simulink model "sepic_2"  (Simulink 7.4)
settings: Solver=ode23tb  StartTime=0.0  StopTime=.01  MaxStep=.01/Fswitch  RelTol=1e-3
InitFcn:
  | clc
  | Fswitch=330e3;
  | Comp_Tau=1e-8;
  | Vset=3.3;
  | Iout=1;
  | Rload=Vset/Iout;
  | Imax=2.5;
  | Iload=Imax-Iout;
  | Tload =5e-3;
  | FET_Ron=8e-3;
  | FET_Snub=1e3;
  | L1=4.6e-6;
  | L1_R = .005;
  | L2=L1;
  | L2_R=L1_R;
  | Cs=10e-6;
  | ESR_cs=.01;
  | Cout=140e-6;
  | ESR_out=4.8e-3;
  | Vfwd_Diode=0.25;
  | R_Diode=0.1;
libraries: powerlib x14, simulink x2, simulink_extras x1
settings Model: Creator=Dick  LastModifiedBy=dbenson  SimulationMode=accelerator
settings SolverCC: SolverResetMethod=Robust

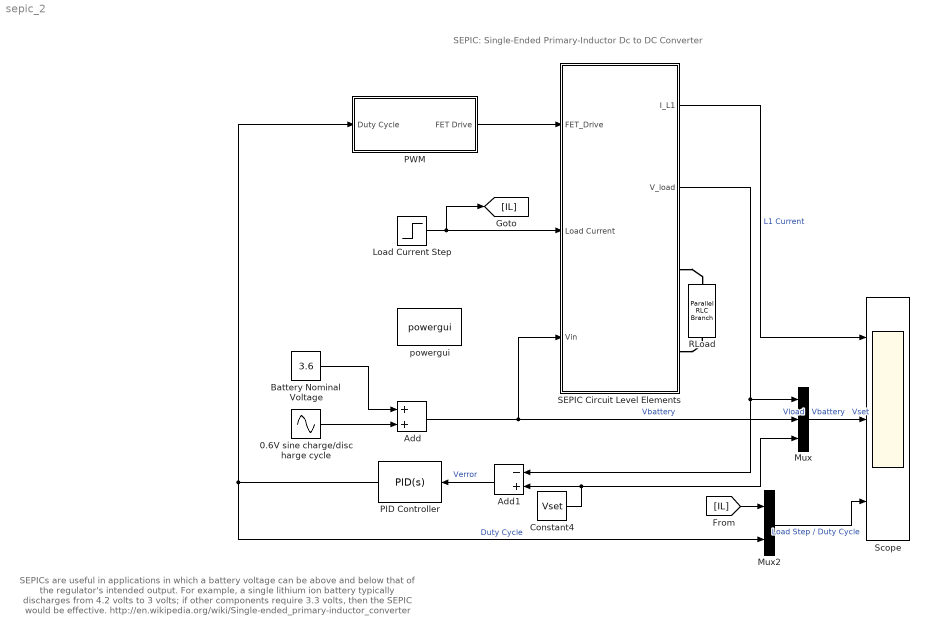
== system sepic_2 ==
  note: SEPICs are useful in applications in which a battery voltage  can be above and below that of the regulator's intended output.
      |  For example, a single lithium ion battery typically discharges from 4.2 volts to 3 volts; if other components require 3.3 volts,
      | then the SEPIC would be effective.
      |
      | http://en.wikipedia.org/wiki/Single-ended_primary-inductor_converter
  note: SEPIC: Single-Ended Primary-Inductor Dc to DC Converter
  0.6V sine charge/discharge cycle : Sin  Amplitude=.6  Bias=0  Frequency=2*pi*100  Phase=0  Samples=10  SampleTime=0  Offset=0
  Add : Sum  OutDataType=fixdt(1, 16)  OutScaling=2^-10
  Add1 : Sum  Inputs=-+  OutDataType=fixdt(1, 16)  OutScaling=2^-10
  Battery Nominal Voltage : Constant  Value=3.6  OutDataType=fixdt(1, 16)  OutScaling=2^0
  Constant4 : Constant  Value=Vset  OutDataType=fixdt(1, 16)  OutScaling=2^0
  Load Current Step : Step  Time=Tload  After=Iload  SampleTime=0
  Mux : Mux  Inputs=3
  Mux2 : Mux  Inputs=2
  PID Controller : simulink/Continuous/PID Controller  DialogController=pidpack.PIDConfig.pidDDGCreate  DialogControllerArgs=DataTag0  SystemSampleTime=-1  Controller=PID  TimeDomain=Continuous-time  SampleTime=1  IntegratorMethod=Forward Euler  FilterMethod=Forward Euler  Form=Parallel  P=.1  I=1000  D=0  N=100  InitialConditionSource=internal  InitialConditionForIntegrator=0  InitialConditionForFilter=0  ExternalReset=none  LimitOutput=off  UpperSaturationLimit=inf  LowerSaturationLimit=-inf  LinearizeAsGain=off  AntiWindupMode=none  Kb=1  TrackingMode=off  Kt=1  PParamMin=[]  PParamMax=[]  IParamMin=[]  IParamMax=[]  DParamMin=[]  DParamMax=[]  NParamMin=[]  NParamMax=[]  KbParamMin=[]  KbParamMax=[]  KtParamMin=[]  KtParamMax=[]  POutMin=[]  POutMax=[]  IOutMin=[]  IOutMax=[]  DOutMin=[]  DOutMax=[]  NOutMin=[]  NOutMax=[]  KbOutMin=[]  KbOutMax=[]  KtOutMin=[]  KtOutMax=[]  IntegratorOutMin=[]  IntegratorOutMax=[]  FilterOutMin=[]  FilterOutMax=[]  SumOutMin=[]  SumOutMax=[]  SumI1OutMin=[]  SumI1OutMax=[]  SumI2OutMin=[]  SumI2OutMax=[]  SumI3OutMin=[]  SumI3OutMax=[]  SumDOutMin=[]  SumDOutMax=[]  SaturationOutMin=[]  SaturationOutMax=[]  IntegratorContinuousStateAttributes=''  IntegratorStateMustResolveToSignalObject=off  IntegratorRTWStateStorageClass=Auto  FilterContinuousStateAttributes=''  FilterStateMustResolveToSignalObject=off  FilterRTWStateStorageClass=Auto
  PWM : Subsystem  mask{Fsw=Fswitch, Tau=Comp_Tau}
      mask prompts: Fsw "Switch Frequency"; Tau "Comparitor Time Constant"
  RLoad : powerlib/Elements/Parallel RLC Branch  DialogController=POWERSYS.PowerSysDialog  PhysicalDomain=powersysdomain  SubClassName=unknown  LeftPortType=p1  RightPortType=p1  LConnTagsString=a  RConnTagsString=__new0  BranchType=R  Resistance=Rload  Inductance=1e-3  SetiL0=off  InitialCurrent=0  Capacitance=1e-6  Setx0=off  InitialVoltage=0  Measurements=None
  SEPIC Circuit Level Elements : Subsystem
  Scope : Scope  NumInputPorts=3
      settings: TimeRange=0.01  YMin=-10~0~-0.3  YMax=10~5~1.7  MaxDataPoints=1e6
  powergui : powerlib/powergui  Priority=1  SystemSampleTime=-1  SimulationMode=Continuous  SampleTime=50e-6  frequency=60  SPID=off  DisableSnubberDevices=off  DisableRonSwitches=off  DisableVfSwitches=off  SwTol=0  Interpol=off  frequencyindice=0  echomessages=off  HookPort=off  DisplayEquations=off  FunctionMessages=off  EnableUseOfTLC=off  x0status=blocks  RestoreLinks=warning  Frange=[0:2:500]  Ylog=off  Xlog=on  ShowGrid=off  save=off  variable=ZData  ZoomFFT=on  StartTime=0.0  cycles=1  DisplayStyle=1  fundamental=60  FreqAxis=off  MaxFrequency=1000  frequencyindicesteady=1  RmsSteady=1  display=off  Ts=0  methode=off
  wires:
  PWM/1(FET Drive) -> SEPIC Circuit Level Elements/1(FET_Drive)
  0.6V sine charge/discharge cycle/1 -> Add/2
  Load Current Step/1 -> SEPIC Circuit Level Elements/2(Load Current), [IL]
  SEPIC Circuit Level Elements/2(V_load) -> Add1/1, Mux/1
  Add1/1 -> PID Controller/1  "Verror"
  Constant4/1 -> Add1/2, Mux/3
  PID Controller/1 -> PWM/1(Duty Cycle), Mux2/2  "Duty Cycle"
  Add/1 -> SEPIC Circuit Level Elements/3(Vin), Mux/2  "Vbattery"
  Battery Nominal Voltage/1 -> Add/1
  Mux/1 -> Scope/2  "Vload   Vbattery   Vset"
  SEPIC Circuit Level Elements/1(I_L1) -> Scope/1  "L1 Current"
  Mux2/1 -> Scope/3  "Load Step / Duty Cycle"
  [IL] -> Mux2/1
  connections:
  SEPIC Circuit Level Elements/RConn1 -- RLoad/LConn1
  SEPIC Circuit Level Elements/RConn2 -- RLoad/RConn1

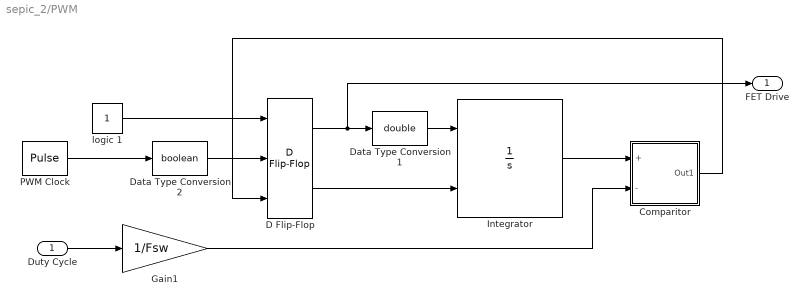
== system sepic_2/PWM ==
  Duty Cycle : Inport  OutDataType=sfix(16)  OutScaling=2^0
  Comparitor : Subsystem
  D Flip-Flop : simulink_extras/Flip Flops/D Flip-Flop  SystemSampleTime=-1
  Data Type Conversion1 : DataTypeConversion  OutDataTypeMode=double  OutDataType=fixdt(1,16,16)  OutDataTypeStr=double  SaturateOnIntegerOverflow=on
  Data Type Conversion2 : DataTypeConversion  OutDataTypeMode=boolean  OutDataType=fixdt(1,16,16)  OutDataTypeStr=boolean  SaturateOnIntegerOverflow=on
  Gain1 : Gain  Gain=1/Fsw  ParameterDataType=fixdt(1, 16)  ParameterScaling=2^0  OutDataType=fixdt(1, 16)  OutScaling=2^0
  Integrator : Integrator  ExternalReset=level
  PWM Clock : DiscretePulseGenerator  PulseType=Time based  Amplitude=1  Period=1/Fsw  PulseWidth=50  PhaseDelay=0  SampleTime=1
  logic 1 : Constant  OutDataTypeMode=boolean  OutDataType=sfix(16)  OutScaling=2^0  OutDataTypeStr=boolean
  FET Drive : Outport  OutDataType=sfix(16)  OutScaling=2^0
  wires:
  D Flip-Flop/2 -> Integrator/2
  logic 1/1 -> D Flip-Flop/1
  Integrator/1 -> Comparitor/1(+)
  D Flip-Flop/1 -> FET Drive/1, Data Type Conversion1/1
  Comparitor/1(Out1) -> D Flip-Flop/3
  Data Type Conversion2/1 -> D Flip-Flop/2
  Data Type Conversion1/1 -> Integrator/1
  Duty Cycle/1 -> Gain1/1
  Gain1/1 -> Comparitor/2(-)
  PWM Clock/1 -> Data Type Conversion2/1

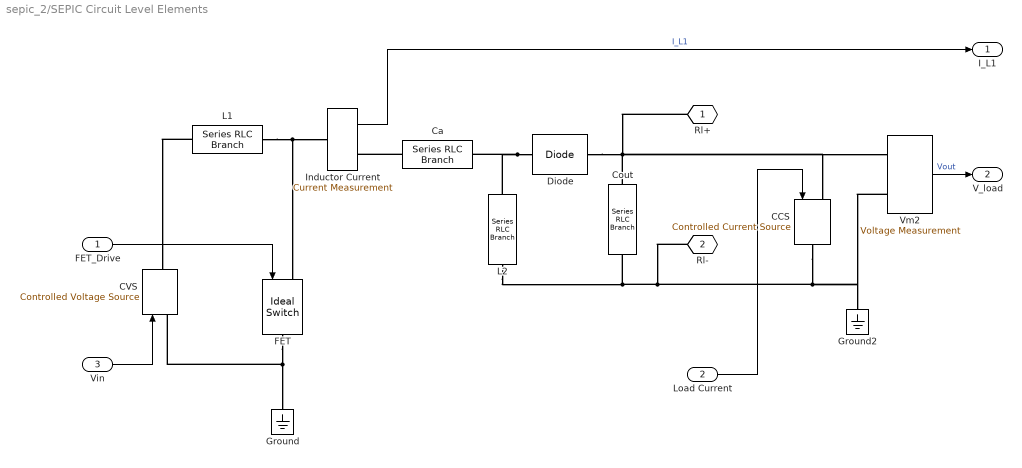
== system sepic_2/SEPIC Circuit Level Elements ==
  FET_Drive : Inport
  Load Current : Inport  Port=2
  Vin : Inport  Port=3
  CCS : powerlib/Electrical Sources/Controlled Current Source  DialogController=POWERSYS.PowerSysDialog  SystemSampleTime=-1  Initialize=on  Source_Type=DC  Amplitude=0  Phase=0  Frequency=0  Measurements=Current
  CVS : powerlib/Electrical Sources/Controlled Voltage Source  DialogController=POWERSYS.PowerSysDialog  SystemSampleTime=-1  Initialize=on  Source_Type=AC  Amplitude=0  Phase=0  Frequency=0  Measurements=None
  Ca : powerlib/Elements/Series RLC Branch  DialogController=POWERSYS.PowerSysDialog  PhysicalDomain=powersysdomain  SubClassName=unknown  LeftPortType=p1  RightPortType=p1  LConnTagsString=__new0  RConnTagsString=__new0  BranchType=RC  Resistance=ESR_cs  Inductance=1e-3  SetiL0=off  InitialCurrent=0  Capacitance=Cs  Setx0=on  InitialVoltage=0  Measurements=None
  Cout : powerlib/Elements/Series RLC Branch  DialogController=POWERSYS.PowerSysDialog  PhysicalDomain=powersysdomain  SubClassName=unknown  LeftPortType=p1  RightPortType=p1  LConnTagsString=__new0  RConnTagsString=__new0  BranchType=RC  Resistance=ESR_out  Inductance=1e-3  SetiL0=off  InitialCurrent=0  Capacitance=Cout  Setx0=on  InitialVoltage=0  Measurements=None
  Diode : powerlib/Power Electronics/Diode  DialogController=POWERSYS.PowerSysDialog  SystemSampleTime=-1  Ron=R_Diode  Lon=0  Vf=Vfwd_Diode  IC=0  UseSnubber=off  Rs=inf  Cs=inf  Measurements=off
  FET : powerlib/Power Electronics/Ideal Switch  DialogController=POWERSYS.PowerSysDialog  SystemSampleTime=-1  Ron=FET_Ron  Lon=0  IC=0  Rs=FET_Snub  Cs=inf  Measurements=off
  Ground : powerlib/Elements/Ground  DialogController=POWERSYS.PowerSysDialog  PhysicalDomain=powersysdomain  SubClassName=unknown  LeftPortType=p1  RightPortType=p1  LConnTagsString=a
  Ground2 : powerlib/Elements/Ground  DialogController=POWERSYS.PowerSysDialog  PhysicalDomain=powersysdomain  SubClassName=unknown  LeftPortType=p1  RightPortType=p1  LConnTagsString=a
  Inductor Current : powerlib/Measurements/Current Measurement  DialogController=POWERSYS.PowerSysDialog  SystemSampleTime=-1  PhasorSimulation=off  OutputType=Complex  PSBequivalent=0
  L1 : powerlib/Elements/Series RLC Branch  DialogController=POWERSYS.PowerSysDialog  PhysicalDomain=powersysdomain  SubClassName=unknown  LeftPortType=p1  RightPortType=p1  LConnTagsString=__new0  RConnTagsString=__new0  BranchType=RL  Resistance=L1_R  Inductance=L1  SetiL0=off  InitialCurrent=0  Capacitance=1e-6  Setx0=off  InitialVoltage=0  Measurements=None
  L2 : powerlib/Elements/Series RLC Branch  DialogController=POWERSYS.PowerSysDialog  PhysicalDomain=powersysdomain  SubClassName=unknown  LeftPortType=p1  RightPortType=p1  LConnTagsString=__new0  RConnTagsString=__new0  BranchType=RL  Resistance=L2_R  Inductance=L2  SetiL0=off  InitialCurrent=0  Capacitance=1e-6  Setx0=off  InitialVoltage=0  Measurements=None
  Vm2 : powerlib/Measurements/Voltage Measurement  DialogController=POWERSYS.PowerSysDialog  SystemSampleTime=-1  PhasorSimulation=off  OutputType=Complex  PSBequivalent=0
  Rl+ : PMIOPort  Tag=PMCPort  Port=1  Side=Right
  Rl- : PMIOPort  Tag=PMCPort  Port=2  Side=Right
  I_L1 : Outport
  V_load : Outport  Port=2
  wires:
  FET_Drive/1 -> FET/1
  Inductor Current/1 -> I_L1/1  "I_L1"
  Vm2/1 -> V_load/1  "Vout"
  Load Current/1 -> CCS/1
  Vin/1 -> CVS/1
  connections:
  Diode/LConn1 -- L2/LConn1 -- Ca/LConn1
  Vm2/LConn2 -- Ground2/LConn1 -- CCS/RConn1 -- Cout/RConn1 -- L2/RConn1 -- Rl-/RConn1
  FET/RConn1 -- Ground/LConn1 -- CVS/LConn1
  L1/LConn1 -- CVS/RConn1
  L1/RConn1 -- FET/LConn1 -- Inductor Current/LConn1
  Ca/RConn1 -- Inductor Current/RConn1
  Vm2/LConn1 -- CCS/LConn1 -- Diode/RConn1 -- Cout/LConn1 -- Rl+/RConn1

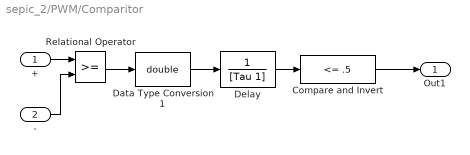
== system sepic_2/PWM/Comparitor ==
  + : Inport  OutDataType=sfix(16)  OutScaling=2^0
  - : Inport  Port=2  OutDataType=sfix(16)  OutScaling=2^0
  "Compare and Invert " : simulink/Logic and Bit Operations/Compare To Constant  SystemSampleTime=-1  relop=<=  const=.5  LogicOutDataTypeMode=boolean  ZeroCross=off
  Data Type Conversion1 : DataTypeConversion  OutDataTypeMode=double  OutDataType=fixdt(1,16,16)  OutDataTypeStr=double  SaturateOnIntegerOverflow=on
  Delay : TransferFcn  Denominator=[Tau 1]
  Relational Operator : RelationalOperator  InputSameDT=on
  Out1 : Outport  OutDataType=sfix(16)  OutScaling=2^0
  wires:
  Relational Operator/1 -> Data Type Conversion1/1
  +/1 -> Relational Operator/1
  Delay/1 -> "Compare and Invert "/1
  -/1 -> Relational Operator/2
  "Compare and Invert "/1 -> Out1/1
  Data Type Conversion1/1 -> Delay/1
